simulink model "dummy_try"  (R2015a)
settings: Solver=ode45  StartTime=0.0  StopTime=100.0  RelTol=1e-3
values from neighbouring files (symbols this model uses):
  Hf_MIMO = modred(Hf_MIMO, elim_state)    [ModelareArchNew.m]    (also in SSModel.m = minreal(Hf_MIMO); incercare0306.m = [Hth Hth; Hthdot(1,1) Hthdot(1,2);            Hps Hps; Hpsdo; try_0805.m; try_checkstuff_BUN.m = ssest(data6, 6, 'Form', 'canonical', Options))
  Hph = tfest(dataPhi, [2 2], [0 0], Options)    [ModelareArchNew.m]    (also in incercare0306.m = Hth; try_0805.m = tfest(dataPhi, [2 2], [2 2], 'Ts', Te))
  Hphdot = tfest(dataPHId, 1, 1, Options)    [ModelareArchNew.m]    (also in incercare0306.m = ssest(dataPHIdV, 1, 'Form', 'canonical', Options); try_0805.m = tfest(dataPHId, 2, 1, Options, 'Ts', 0.01, 'Feedthrough', tr)
  Hps = tfest(dataPSI, [3 3], [1 1], Options)    [ModelareArchNew.m]    (also in incercare0306.m = Hth; try_0805.m = tfest(dataPSI, [2 2], [1 1], 'Ts', Te))
  Hpsdot = tfest(dataPSdot, 1, 1, Options)    [ModelareArchNew.m]    (also in incercare0306.m = n4sid(dataPSdotV, 3, 'Form', 'canonical', 'Ts', 0, Options); try_0805.m = idtf(Hpsdot))
  Hth = tfest(dataTH, [2 2], [1 1], Options)    [ModelareArchNew.m]    (also in SSModel.m = n4sid(dataTH, 1, 'Ts', 0, Options); incercare0306.m = ss(Hth); try_0805.m = tfest(dataTH, [2 2], [2 2], 'Ts', Te))
  Hthdot = tfest(dataTHdot, 1, 1, Options)    [ModelareArchNew.m]    (also in SSModel.m = Hth*D; incercare0306.m = n4sid(dataTHdotV, 3, 'Form', 'canonical', 'Ts', 0, Options); try_0805.m = idtf(Hthdot))
  K = lqr(Hf_MIMO.a, Hf_MIMO.b, Q, R)    [ModelareArchNew.m]    (also in SSModel.m; lqrbun.mat = [-0.0544920986643  -0.0223334040175  -2.47238623528  -0.3309; try_0805.m; try_checkstuff_BUN.m = K/10)
  Te = l.T0    [ModelareArchNew.m]    (also in SSModel.m; incercare0306.m; try_0805.m = t(2)-t(1); try_checkstuff_BUN.m = 0.003)
libraries: simulink x4
settings Model: Creator=Maria  LastModifiedBy=Maria

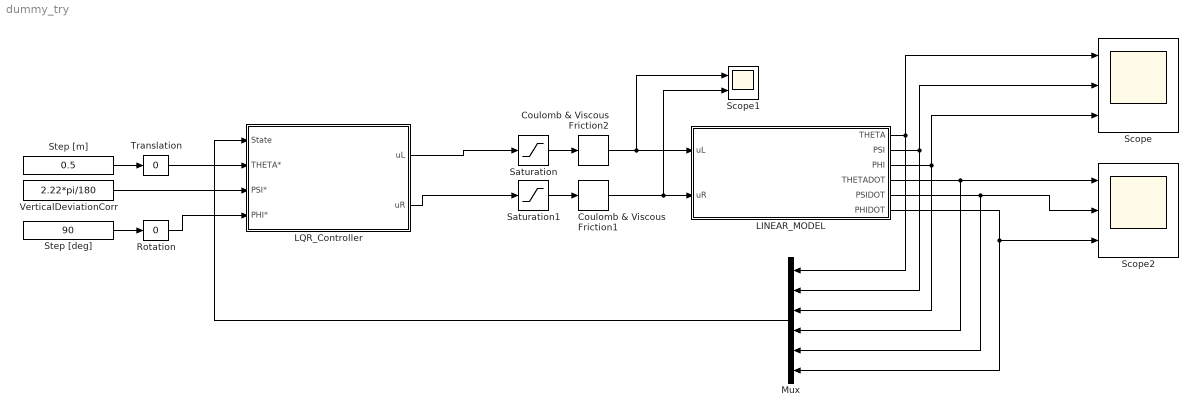
== system dummy_try ==
  Coulomb & Viscous Friction1 : simulink/Discontinuities/Coulomb & Viscous Friction  offset=0.055  gain=1
  Coulomb & Viscous Friction2 : simulink/Discontinuities/Coulomb & Viscous Friction  offset=0.055  gain=1
  "LINEAR_MODEL " : Subsystem
  "LQR_Controller " : Subsystem
  Mux : Mux  Inputs=6
  Rotation : simulink/Math Operations/Slider Gain  low=-5  gain=0  high=5
  Saturation : Saturate  UpperLimit=0.7  LowerLimit=-0.7
  Saturation1 : Saturate  UpperLimit=0.7  LowerLimit=-0.7
  Scope : Scope  NumInputPorts=3
      settings: TickLabels=on  YMin=-5~-5~-5  YMax=5~5~5
  Scope1 : Scope  NumInputPorts=2
      settings: YMin=-5~-5  YMax=5~5
  Scope2 : Scope  NumInputPorts=3
      settings: YMin=-5~-5~-5  YMax=5~5~5  SaveName=ScopeData2
  Step [deg] : Constant  Value=90
  Step [m] : Constant  Value=0.5
  Translation : simulink/Math Operations/Slider Gain  low=-5  gain=0  high=5
  "VerticalDeviationCorr " : Constant  Value=2.22*pi/180
  wires:
  "LINEAR_MODEL "/2("PSI ") -> Scope/2, Mux/2
  "LINEAR_MODEL "/4("THETADOT ") -> Mux/4, Scope2/1
  "LINEAR_MODEL "/5("PSIDOT ") -> Mux/5, Scope2/2
  "LINEAR_MODEL "/6("PHIDOT ") -> Mux/6, Scope2/3
  Mux/1 -> "LQR_Controller "/1("State ")
  Saturation/1 -> Coulomb & Viscous Friction2/1
  Saturation1/1 -> Coulomb & Viscous Friction1/1
  "VerticalDeviationCorr "/1 -> "LQR_Controller "/3("PSI* ")
  Rotation/1 -> "LQR_Controller "/4("PHI* ")
  "LQR_Controller "/1("uL ") -> Saturation/1
  "LQR_Controller "/2("uR ") -> Saturation1/1
  Translation/1 -> "LQR_Controller "/2(THETA*)
  Step [m]/1 -> Translation/1
  Step [deg]/1 -> Rotation/1
  "LINEAR_MODEL "/1("THETA ") -> Scope/1, Mux/1
  "LINEAR_MODEL "/3("PHI ") -> Scope/3, Mux/3
  Coulomb & Viscous Friction2/1 -> Scope1/1, "LINEAR_MODEL "/1("uL ")
  Coulomb & Viscous Friction1/1 -> Scope1/2, "LINEAR_MODEL "/2("uR ")

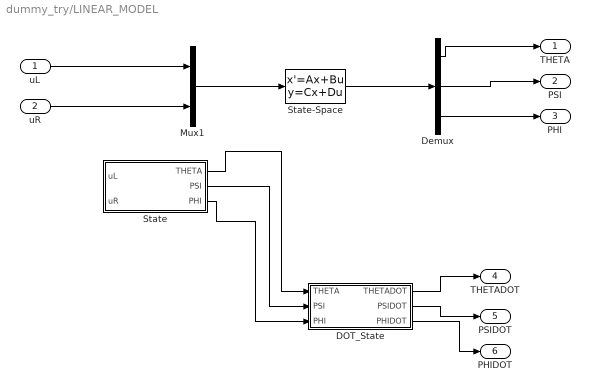
== system dummy_try/LINEAR_MODEL  ==
  "uL " : Inport
  "uR " : Inport  Port=2
  "DOT_State " : Subsystem
  Demux : Demux  Outputs=3
  Mux1 : Mux  Inputs=2
  "State " : Subsystem
  State-Space : StateSpace  A=Hf_MIMO.a  B=Hf_MIMO.b  C=Hf_MIMO.c  D=Hf_MIMO.d  X0=0
  "THETA " : Outport
  "PSI " : Outport  Port=2
  "PHI " : Outport  Port=3
  "THETADOT " : Outport  Port=4
  "PSIDOT " : Outport  Port=5
  "PHIDOT " : Outport  Port=6
  wires:
  "State "/1("THETA ") -> "DOT_State "/1("THETA ")
  "State "/2("PSI ") -> "DOT_State "/2(PSI)
  "State "/3("PHI ") -> "DOT_State "/3("PHI ")
  Mux1/1 -> State-Space/1
  "uL "/1 -> Mux1/1
  "uR "/1 -> Mux1/2
  State-Space/1 -> Demux/1
  Demux/1 -> "THETA "/1
  Demux/2 -> "PSI "/1
  Demux/3 -> "PHI "/1
  "DOT_State "/1("THETADOT ") -> "THETADOT "/1
  "DOT_State "/2("PSIDOT ") -> "PSIDOT "/1
  "DOT_State "/3("PHIDOT ") -> "PHIDOT "/1

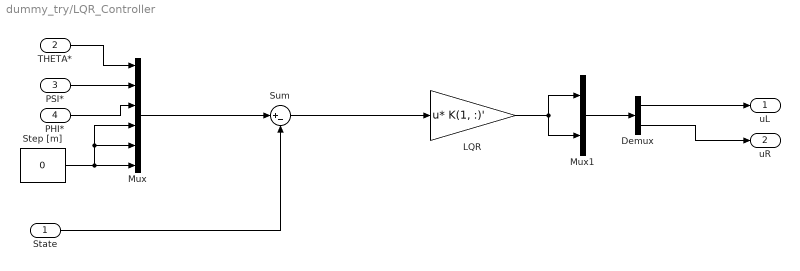
== system dummy_try/LQR_Controller  ==
  "State " : Inport
  THETA* : Inport  Port=2
  "PSI* " : Inport  Port=3
  "PHI* " : Inport  Port=4
  Demux : Demux  Outputs=2
  LQR : Gain  Gain=K(1, :)'  Multiplication=Matrix(u*K)
  Mux : Mux  Inputs=6
  Mux1 : Mux  Inputs=2
  Step [m] : Constant  Value=0
  Sum : Sum  Inputs=|+-
  "uL " : Outport
  "uR " : Outport  Port=2
  wires:
  THETA*/1 -> Mux/1
  "PSI* "/1 -> Mux/2
  "PHI* "/1 -> Mux/3
  Mux/1 -> Sum/1
  Sum/1 -> LQR/1
  Demux/1 -> "uL "/1
  Demux/2 -> "uR "/1
  "State "/1 -> Sum/2
  Mux1/1 -> Demux/1
  LQR/1 -> Mux1/2, Mux1/1
  Step [m]/1 -> Mux/4, Mux/5, Mux/6

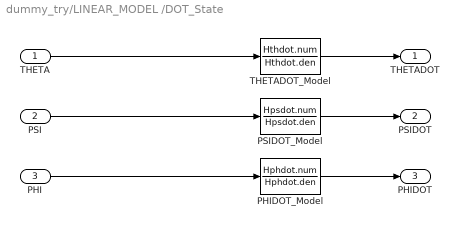
== system dummy_try/LINEAR_MODEL /DOT_State  ==
  "THETA " : Inport
  PSI : Inport  Port=2
  "PHI " : Inport  Port=3
  "PHIDOT_Model " : DiscreteFilter  Numerator=Hphdot.num  Denominator=Hphdot.den  SampleTime=Te
  "PSIDOT_Model " : DiscreteFilter  Numerator=Hpsdot.num  Denominator=Hpsdot.den  SampleTime=Te
  "THETADOT_Model " : DiscreteFilter  Numerator=Hthdot.num  Denominator=Hthdot.den  SampleTime=Te
  "THETADOT " : Outport
  "PSIDOT " : Outport  Port=2
  "PHIDOT " : Outport  Port=3
  wires:
  "THETADOT_Model "/1 -> "THETADOT "/1
  "PSIDOT_Model "/1 -> "PSIDOT "/1
  "PHIDOT_Model "/1 -> "PHIDOT "/1
  "PHI "/1 -> "PHIDOT_Model "/1
  PSI/1 -> "PSIDOT_Model "/1
  "THETA "/1 -> "THETADOT_Model "/1

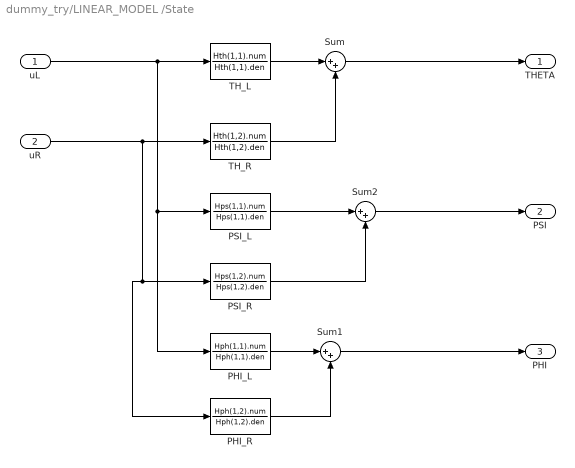
== system dummy_try/LINEAR_MODEL /State  ==
  "uL " : Inport
  "uR " : Inport  Port=2
  "PHI_L " : TransferFcn  Numerator=Hph(1,1).num  Denominator=Hph(1,1).den
  "PHI_R " : TransferFcn  Numerator=Hph(1,2).num  Denominator=Hph(1,2).den
  "PSI_L " : TransferFcn  Numerator=Hps(1,1).num  Denominator=Hps(1,1).den
  "PSI_R " : TransferFcn  Numerator=Hps(1,2).num  Denominator=Hps(1,2).den
  Sum : Sum  Inputs=|++
  Sum1 : Sum  Inputs=|++
  Sum2 : Sum  Inputs=|++
  "TH_L " : TransferFcn  Numerator=Hth(1,1).num  Denominator=Hth(1,1).den
  "TH_R " : TransferFcn  Numerator=Hth(1,2).num  Denominator=Hth(1,2).den
  "THETA " : Outport
  "PSI " : Outport  Port=2
  "PHI " : Outport  Port=3
  wires:
  "uL "/1 -> "TH_L "/1, "PHI_L "/1, "PSI_L "/1
  "uR "/1 -> "TH_R "/1, "PHI_R "/1, "PSI_R "/1
  Sum/1 -> "THETA "/1
  "TH_L "/1 -> Sum/1
  "TH_R "/1 -> Sum/2
  "PHI_L "/1 -> Sum1/1
  Sum1/1 -> "PHI "/1
  "PHI_R "/1 -> Sum1/2
  "PSI_L "/1 -> Sum2/1
  Sum2/1 -> "PSI "/1
  "PSI_R "/1 -> Sum2/2
